simulink model "debug_FTExternalForces_legacy"  (Simulink 8.3)
settings: Solver=FixedStepDiscrete  StartTime=0.0  StopTime=inf  FixedStep=0.01  RelTol=1e-3
InitFcn:
  | ROBOT_DOF=23;
libraries: WBToolboxLibrary x7
settings Model: Creator=DanielePucci  LastModifiedBy=gnava  CovSFcnEnable=on
settings DataIOCC: SaveFormat=StructureWithTime  SignalLoggingSaveFormat=Dataset
settings DebuggingCC: UnderspecifiedInitializationDetection=Simplified  MergeDetectMultiDrivingBlocksExec=error  SolverPrmCheckMsg=none  FrameProcessingCompatibilityMsg=error  StateNameClashWarn=none
settings HardwareCC: ProdBitPerPointer=64  ProdLargestAtomicFloat=Float  ProdIntDivRoundTo=Zero  ProdEndianess=LittleEndian  ProdHWDeviceType=Specified
settings GRTTargetCC: GeneratePreprocessorConditionals=Use local settings  CombineOutputUpdateFcns=on  GRTInterface=off

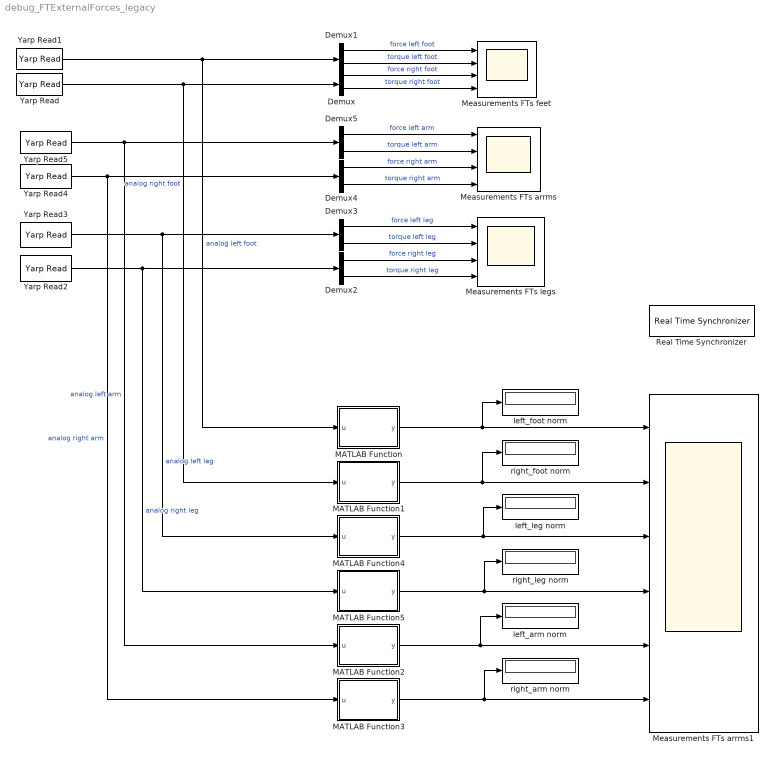
== system debug_FTExternalForces_legacy ==
  Demux{,1..5} (6 alike) : Demux  Outputs=2
  MATLAB Function : MATLAB Function  TreatAsAtomicUnit=on
      settings: PermitHierarchicalResolution=ParametersOnly
  MATLAB Function1 : MATLAB Function  TreatAsAtomicUnit=on
      settings: PermitHierarchicalResolution=ParametersOnly
  MATLAB Function2 : MATLAB Function  TreatAsAtomicUnit=on
      settings: PermitHierarchicalResolution=ParametersOnly
  MATLAB Function3 : MATLAB Function  TreatAsAtomicUnit=on
      settings: PermitHierarchicalResolution=ParametersOnly
  MATLAB Function4 : MATLAB Function  TreatAsAtomicUnit=on
      settings: PermitHierarchicalResolution=ParametersOnly
  MATLAB Function5 : MATLAB Function  TreatAsAtomicUnit=on
      settings: PermitHierarchicalResolution=ParametersOnly
  Measurements FTs arrms : Scope  NumInputPorts=4
      settings: TimeRange=60  MaxDataPoints=5000  SaveToWorkspace=off  YMin=-0.82779~-0.02821~-1.24939~-0.03433  YMax=1.09268~0.03263~1.11267~0.0343  SampleTime=-1
  Measurements FTs arrms1 : Scope  NumInputPorts=6
      settings: TimeRange=60  MaxDataPoints=5000  SaveToWorkspace=off  YMin=-0.82779~-0.02821~-1.24939~-0.03433~-5~-5  YMax=1.09268~0.03263~1.11267~0.0343~5~5  SampleTime=-1
  Measurements FTs feet : Scope  NumInputPorts=4
      settings: TimeRange=60  ShowLegends=on  MaxDataPoints=5000  SaveToWorkspace=off  YMin=-9.66328~-0.48787~-57.09767~-2.05544  YMax=53.98887~0.44951~-22.56265~3.67473  SampleTime=-1
  Measurements FTs legs : Scope  NumInputPorts=4
      settings: TimeRange=60  ShowLegends=on  MaxDataPoints=5000  SaveToWorkspace=off  YMin=-23.57964~-8.18457~-44.53745~-6.86801  YMax=37.68669~8.35653~36.21183~8.53448  SampleTime=-1
  Real Time Synchronizer : WBToolboxLibrary/Utilities/Real Time Synchronizer  period=0.01
  Yarp Read : WBToolboxLibrary/Utilities/Yarp Read  portName='/icub/right_foot/analog:o'  signalSize=6  timeout=0.5  blocking=off  timestamp=off  autoconnect=on  errorOnConnection=off
  Yarp Read1 : WBToolboxLibrary/Utilities/Yarp Read  portName='/icub/left_foot/analog:o'  signalSize=6  timeout=0.5  blocking=off  timestamp=off  autoconnect=on  errorOnConnection=off
  Yarp Read2 : WBToolboxLibrary/Utilities/Yarp Read  portName='/icub/right_leg/analog:o'  signalSize=6  timeout=0.5  blocking=off  timestamp=off  autoconnect=on  errorOnConnection=off
  Yarp Read3 : WBToolboxLibrary/Utilities/Yarp Read  portName='/icub/left_leg/analog:o'  signalSize=6  timeout=0.5  blocking=off  timestamp=off  autoconnect=on  errorOnConnection=off
  Yarp Read4 : WBToolboxLibrary/Utilities/Yarp Read  portName='/icub/right_arm/analog:o'  signalSize=6  timeout=0.5  blocking=off  timestamp=off  autoconnect=on  errorOnConnection=off
  Yarp Read5 : WBToolboxLibrary/Utilities/Yarp Read  portName='/icub/left_arm/analog:o'  signalSize=6  timeout=0.5  blocking=off  timestamp=off  autoconnect=on  errorOnConnection=off
  left_arm norm : Display
  left_foot norm : Display
  left_leg norm : Display
  right_arm norm : Display
  right_foot norm : Display
  right_leg norm : Display
  wires:
  Yarp Read/1 -> Demux/1, MATLAB Function1/1(u)  "analog right foot"
  Demux/1 -> Measurements FTs feet/3  "force right foot"
  Demux/2 -> Measurements FTs feet/4  "torque right foot"
  Yarp Read1/1 -> Demux1/1, MATLAB Function/1(u)  "analog left foot"
  Demux1/1 -> Measurements FTs feet/1  "force left foot"
  Demux1/2 -> Measurements FTs feet/2  "torque left foot"
  Yarp Read2/1 -> Demux2/1, MATLAB Function5/1(u)  "analog right leg"
  Demux2/1 -> Measurements FTs legs/3  "force right leg"
  Demux2/2 -> Measurements FTs legs/4  "torque right leg"
  Yarp Read3/1 -> Demux3/1, MATLAB Function4/1(u)  "analog left leg"
  Demux3/1 -> Measurements FTs legs/1  "force left leg"
  Demux3/2 -> Measurements FTs legs/2  "torque left leg"
  Yarp Read4/1 -> Demux4/1, MATLAB Function3/1(u)  "analog right arm"
  Demux4/1 -> Measurements FTs arrms/3  "force right arm"
  Demux4/2 -> Measurements FTs arrms/4  "torque right arm"
  Yarp Read5/1 -> Demux5/1, MATLAB Function2/1(u)  "analog left arm"
  Demux5/1 -> Measurements FTs arrms/1  "force left arm"
  Demux5/2 -> Measurements FTs arrms/2  "torque left arm"
  MATLAB Function1/1(y) -> right_foot norm/1, Measurements FTs arrms1/2
  MATLAB Function4/1(y) -> left_leg norm/1, Measurements FTs arrms1/3
  MATLAB Function5/1(y) -> right_leg norm/1, Measurements FTs arrms1/4
  MATLAB Function2/1(y) -> left_arm norm/1, Measurements FTs arrms1/5
  MATLAB Function3/1(y) -> right_arm norm/1, Measurements FTs arrms1/6
  MATLAB Function/1(y) -> left_foot norm/1, Measurements FTs arrms1/1

== matlab function MATLAB Function1 ==
  data: u input double; y output double
function y = fcn(u)
y =norm(u);

== matlab function MATLAB Function ==
  data: u input double; y output double
function y = fcn(u)
y =norm(u);

== matlab function MATLAB Function2 ==
  data: u input double; y output double
function y = fcn(u)
y =norm(u);

== matlab function MATLAB Function3 ==
  data: u input double; y output double
function y = fcn(u)
y =norm(u);

== matlab function MATLAB Function4 ==
  data: u input double; y output double
function y = fcn(u)
y =norm(u);

== matlab function MATLAB Function5 ==
  data: u input double; y output double
function y = fcn(u)
y =norm(u);
